simulink model "ACDCMG_sim8"  (R2019b)
settings: Solver=ode8  StartTime=0.0  StopTime=0.5  FixedStep=40e-6  MaxStep=1e-2  RelTol=1e-3
InitFcn:
  | Set_parameters_R2018
undefined symbols (not defined in the file): D1, Delta, dis11, dis12, dis2, dis3, dis4, dis5, dis6, DiscIntNeverNeededParam, fn, Fnom, Ion, Lithium, max_min, P_Load_3, Pnom_T1, Pnom_T2, Pnom_T3, Ql_Load_3, R_Load_9, R_Load_DC, Rl, Rls, Ts, Ts_Control, Ts_Power, Ts_PV, V1_LL_T3, Vmin_mppt, VnInv, Vnom_DC, Vnom_Diesel, Vnom_prim, Vnom_sec, Vnom_ter_AC_DC, Xl, Xls
libraries: powerlib x133, powerlib_meascontrol x67, rtlab x23, simulink x7, powerlib_extras x5, electricdrivelib x1, eeSinusoidalMeasurementV2 x1, re_lib x1
(part 5 of 5)

== system ACDCMG_sim8/SM_Grid_Simulation/Grid Bi-directional Converter 1.1 300 (DC) // 150 V (AC) P_nom 3kW2/Control of Inverter/MI Controller/Subsystem ==
  sin_cos : Inport  PortDimensions=2
  Demux : Demux  Outputs=2
  Fcn2 : Fcn  Expr=1*u[1]
  Fcn4 : Fcn  Expr=1*u[3]
  Fcn5 : Fcn  Expr=1*u[5]
  K1 : Constant  Value=0.5
  K2 : Constant  Value=sqrt(3)/2
  Mux2 : Mux  Inputs=6
  Product{,1..3} (4 alike) : Product  SaturateOnIntegerOverflow=on  InputSameDT=on  OutDataTypeStr=Inherit: Same as first input
  Sum : Sum  Inputs=--  SaturateOnIntegerOverflow=on  InputSameDT=on  OutDataTypeStr=Inherit: Same as first input
  Sum1 : Sum  Inputs=-+  SaturateOnIntegerOverflow=on  InputSameDT=on  OutDataTypeStr=Inherit: Same as first input
  Sum2 : Sum  Inputs=--  SaturateOnIntegerOverflow=on  InputSameDT=on  OutDataTypeStr=Inherit: Same as first input
  Sum3 : Sum  Inputs=--  SaturateOnIntegerOverflow=on  InputSameDT=on  OutDataTypeStr=Inherit: Same as first input
  Va : Outport  VectorParamsAs1DForOutWhenUnconnected=off
  Vb : Outport  Port=2  VectorParamsAs1DForOutWhenUnconnected=off
  Vc : Outport  Port=3  VectorParamsAs1DForOutWhenUnconnected=off
  wires:
  sin_cos/1 -> Demux/1
  Demux/1 -> Product/1, Product2/1, Sum2/2, Mux2/1  "sin(wt)"
  Product/1 -> Sum/1
  Product1/1 -> Sum/2
  Product3/1 -> Sum1/1
  Product2/1 -> Sum1/2
  Sum3/1 -> Mux2/6  "cos(wt+2pi/3)"
  Sum2/1 -> Mux2/5  "sin(wt+2pi/3)"
  K1/1 -> Product/2, Product3/2
  K2/1 -> Product1/2, Product2/2
  Sum/1 -> Mux2/3, Sum2/1  "sin(wt-2pi/3)"
  Sum1/1 -> Mux2/4, Sum3/1  "cos(wt-2pi/3)"
  Demux/2 -> Sum3/2, Product3/1, Product1/1, Mux2/2  "cos(wt)"
  Mux2/1 -> Fcn2/1, Fcn4/1, Fcn5/1
  Fcn2/1 -> Va/1
  Fcn4/1 -> Vb/1
  Fcn5/1 -> Vc/1

== system ACDCMG_sim8/SM_Grid_Simulation/Grid Bi-directional Converter 1.1 300 (DC) // 150 V (AC) P_nom 3kW2/Control of Inverter/MI Controller/Subsystem1 ==
  note: AC to DC
  note: DC to AC
  Constant1 : Constant  Value=max_min
  Constant2 : Constant  Value=2*pi
  Deg->Rad : Gain  Gain=pi/180  SaturateOnIntegerOverflow=on  OutDataTypeStr=Inherit: Same as input  ParamDataTypeStr=Inherit: Same as input
  Freq1 : Constant  Value=Fnom
  Freq2 : Constant  Value=2*pi
  Math Function : Math  Operator=mod  SaturateOnIntegerOverflow=on
  Mux5 : Mux  Inputs=2
  OP_max1 : Constant  Value=0
  OP_min1 : Constant  Value=228
  Product7 : Product  Inputs=***  SaturateOnIntegerOverflow=on  InputSameDT=on  OutDataTypeStr=Inherit: Same as first input
  Sum : Sum  SaturateOnIntegerOverflow=on  InputSameDT=on  OutDataTypeStr=Inherit: Same as first input
  Switch2 : Switch  Criteria=u2 > Threshold
  Trigonometric Function : Trigonometry
  Trigonometric Function1 : Trigonometry  Operator=cos
  t : DigitalClock  SampleTime=Ts
  Frec : Outport  VectorParamsAs1DForOutWhenUnconnected=off
  sin_cos : Outport  Port=2  VectorParamsAs1DForOutWhenUnconnected=off
  wt : Outport  Port=3  VectorParamsAs1DForOutWhenUnconnected=off
  wires:
  Switch2/1 -> Deg->Rad/1
  Deg->Rad/1 -> Sum/2
  Freq1/1 -> Frec/1, Product7/1
  Trigonometric Function/1 -> Mux5/1
  Sum/1 -> Math Function/1
  Trigonometric Function1/1 -> Mux5/2
  Product7/1 -> Sum/1
  Freq2/1 -> Product7/3
  Constant2/1 -> Math Function/2
  t/1 -> Product7/2
  Math Function/1 -> wt/1, Trigonometric Function1/1, Trigonometric Function/1
  Mux5/1 -> sin_cos/1
  Constant1/1 -> Switch2/2
  OP_max1/1 -> Switch2/1
  OP_min1/1 -> Switch2/3

== system ACDCMG_sim8/SM_Grid_Simulation/Inverter 300 (DC) // 150 V (AC) P_nom 10 kW4/Control of Inverter/Subsystem2/Subsystem1 ==
  note: Iq* = 2/3*( P*Vq - Q*Vd ) / ( Vd^2 + Vq^2 )
  note: Reference computation:
  note: Id* = 2/3* ( P*Vd + Q*Vq ) / ( Vd^2 + Vq^2 )
  P_ref : Inport  PortDimensions=1
  Q_ref : Inport  Port=2  PortDimensions=1
  Vd : Inport  Port=3  PortDimensions=1
  Vq : Inport  Port=4  PortDimensions=1
  Constant1 : Constant  Commented=on  Value=0
  Demux3 : Demux  Outputs=2
  Fcn3 : Fcn  Expr=u(1)*u(1)+u(2)*u(2)
  Gain : Gain  Gain=2/3
  Mux1 : Mux  Inputs=2
  Mux3 : Mux  Inputs=2
  Product{2..5} (4 alike) : Product  SaturateOnIntegerOverflow=on  InputSameDT=on  OutDataTypeStr=Inherit: Same as first input
  Product6 : Product  Inputs=*/  SaturateOnIntegerOverflow=on  InputSameDT=on  OutDataTypeStr=Inherit: Same as first input
  Scope3 : Scope  NumInputPorts=2
  Sum : Sum  SaturateOnIntegerOverflow=on  InputSameDT=on  OutDataTypeStr=Inherit: Same as first input
  Sum1 : Sum  Inputs=+-  SaturateOnIntegerOverflow=on  InputSameDT=on  OutDataTypeStr=Inherit: Same as first input
  Terminator : Terminator  Commented=on
  Id_ref : Outport
  Iq_ref : Outport  Port=2
  wires:
  Vq/1 -> Mux1/2, Product4/2, Product3/1
  Demux3/1 -> Scope3/1, Id_ref/1
  Mux1/1 -> Fcn3/1
  Product3/1 -> Sum/2
  Mux3/1 -> Gain/1
  Vd/1 -> Mux1/1, Product5/2, Product2/1
  Product4/1 -> Sum1/1
  Product6/1 -> Demux3/1
  Fcn3/1 -> Product6/2
  Demux3/2 -> Scope3/2, Iq_ref/1
  P_ref/1 -> Product2/2, Product4/1
  Gain/1 -> Product6/1
  Product2/1 -> Sum/1
  Q_ref/1 -> Product5/1, Product3/2
  Sum1/1 -> Mux3/2
  Product5/1 -> Sum1/2
  Sum/1 -> Mux3/1

== system ACDCMG_sim8/SM_Grid_Simulation/Inverter 300 (DC) // 150 V (AC) P_nom 10 kW4/Control of Inverter/Subsystem2/WL ==
  In1 : Inport
  freq : Inport  Port=2
  L : Inport  Port=3
  2pai : Constant  Value=2*pi
  Product : Product  Inputs=**
  Product1 : Product  Inputs=***
  Out1 : Outport
  wires:
  2pai/1 -> Product/2
  L/1 -> Product1/3
  freq/1 -> Product/1
  Product1/1 -> Out1/1
  Product/1 -> Product1/2
  In1/1 -> Product1/1

== system ACDCMG_sim8/SM_Grid_Simulation/Inverter 300 (DC) // 150 V (AC) P_nom 10 kW4/Control of Inverter/Subsystem2/WL1 ==
  In1 : Inport
  freq : Inport  Port=2
  L : Inport  Port=3
  2pai : Constant  Value=2*pi
  Product : Product
  Product1 : Product  Inputs=3
  Out1 : Outport
  wires:
  2pai/1 -> Product/2
  L/1 -> Product1/3
  freq/1 -> Product/1
  Product1/1 -> Out1/1
  Product/1 -> Product1/2
  In1/1 -> Product1/1
